simulink model "TEMPLE_COUNTER"  (R2024a)
settings: Solver=FixedStepAuto  StartTime=0.0  StopTime=10.0  FixedStep=0.1  RelTol=1e-3
libraries: simulink x2
settings Model: Creator=prabo  LastModifiedBy=prabo

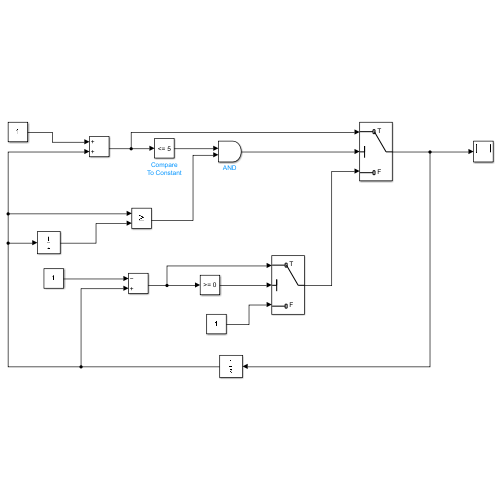
[thumbnail: Simulink's stored preview of the top-level diagram]
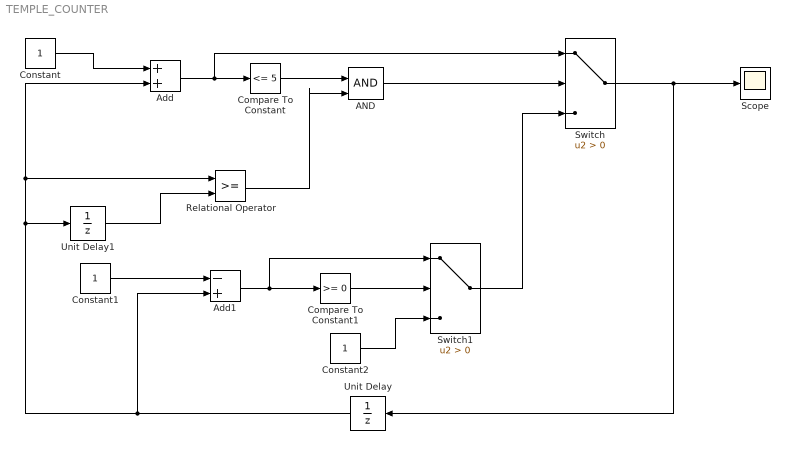
== system TEMPLE_COUNTER ==
  AND : Logic  IconShape=distinctive  AllPortsSameDT=off  OutDataTypeStr=boolean
  Add : Sum
  Add1 : Sum  Inputs=-+
  Compare To Constant : simulink/Logic and Bit Operations/Compare To Constant  relop=<=  const=5  OutDataTypeStr=boolean
  Compare To Constant1 : simulink/Logic and Bit Operations/Compare To Constant  relop=>=  const=0  OutDataTypeStr=boolean
  Constant : Constant
  Constant1 : Constant
  Constant2 : Constant
  Relational Operator : RelationalOperator  OutDataTypeStr=boolean  RndMeth=Simplest  InputSameDT=off
  Scope : Scope
  Switch : Switch  Criteria=u2 > Threshold  SaturateOnIntegerOverflow=off  InputSameDT=off
  Switch1 : Switch  Criteria=u2 > Threshold  SaturateOnIntegerOverflow=off  InputSameDT=off
  Unit Delay : UnitDelay  InitialCondition=-1  SampleTime=-1  HasFrameUpgradeWarning=on
  Unit Delay1 : UnitDelay  InitialCondition=-2  SampleTime=-1  HasFrameUpgradeWarning=on
  wires:
  Switch/1 -> Scope/1, Unit Delay/1
  Switch1/1 -> Switch/3
  Constant/1 -> Add/1
  Unit Delay/1 -> Add1/2, Unit Delay1/1, Relational Operator/1, Add/2
  Compare To Constant/1 -> AND/1
  Add/1 -> Switch/1, Compare To Constant/1
  AND/1 -> Switch/2
  Relational Operator/1 -> AND/2
  Unit Delay1/1 -> Relational Operator/2
  Compare To Constant1/1 -> Switch1/2
  Constant2/1 -> Switch1/3
  Add1/1 -> Switch1/1, Compare To Constant1/1
  Constant1/1 -> Add1/1
